simulink library "adeye_lib"  (R2019a)
settings: Solver=VariableStepAuto  StartTime=0.0  StopTime=10.0  RelTol=1e-3
undefined symbols (not defined in the file): AngularVelocity, Clock_, Data, Data_SL_Info, DiscIntNeverNeededParam, Encoding, Encoding_SL_Info, Header, Height, LinearAcceleration, Orientation, Pose, Step, Twist, Width
libraries: robotlib x47, $bdroot x46, simulink_extras x12, dspsrcs4 x6, dspindex x6, robotcorelib x2, aerolibutil x2, PreScanSimulinkLibrary x1
(part 1 of 4)
settings Model: Creator=adeye  LastModifiedBy=adeye

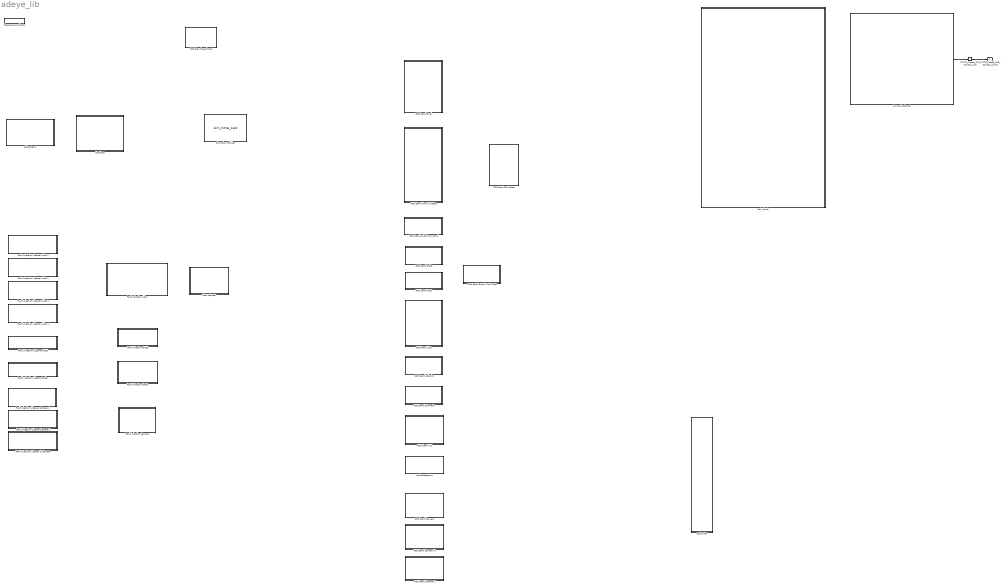
== system adeye_lib ==
  Car_Pose : Subsystem
      mask Display:
      | fprintf('Car_pose\nAdapter\n')
      | 
      | port_label('input',1,'x[m]')
      | port_label('input',2,'y[m]')
      | port_label('input',3,'z[m]')
      | port_label('input',4,'Rotx[deg]')
      | port_label('input',5,'Roty[deg]')
      | port_label('input',6,'Rotz[deg]')
      | port_label('input',7,'CoG Offset(x)')
      | port_label('input',8,'CoG Offset(y)')
      | port_label('input',9,'CoG Offset(z)')
      | 
      | port_label('output',1,'base_link_pose')
  Dynamics_Empty : Subsystem  Tag=Dynamics_Empty
  Fault Injection Camera : Subsystem  mask{idy=200, idx=100, x=100, y=150, R=0, G=0, B=0}
      mask prompts: idy "X"; idx "Y"
      mask DialogControl ParameterGroupVar Prompt: Offset
      mask DialogControl Container3 Prompt: Size
      mask DialogControl Container4 Prompt: Error
      mask Display:
      | fprintf('Fault inj\n Camera\n')
      | 
      | port_label('input',1,'R')
      | port_label('input',2,'G')
      | port_label('input',3,'B')
      | port_label('input',4,'On/Patch')
      | port_label('input',5,'patch/start_x')
      | port_label('input',6,'patch/start_y')
      | port_label('input',7,'patch/size_x')
      | port_label('input',8,'patch/size_y')
      | port_label('input',9,'patch/R')
      | port_label('input',10,'patch/G')
      | port_label('input',11,'patch/B')
      | 
      | port_label('output',1,'R')
      | port_label('output',2,'G')
      | port_label('output',3,'B')
  Fault Injection GNSS : Subsystem  mask{f=20}
      mask prompts: f "Frequency"
      mask Display:
      | fprintf('Fault inj\n GNSS\n')
      | 
      | port_label('input',1,'Pose')
      | port_label('input',2,'On/Off')
      | port_label('input',3,'noise_variance')
      | 
      | port_label('output',1,'Pose')
  Fault Injection Lidar : Subsystem  mask{f=20, p=225*16}
      mask prompts: f "Frequency"; p "Number of detection points"
      mask Display:
      | fprintf('Fault inj\n Lidar\n')
      | 
      | port_label('input',1,'Range[m]')
      | port_label('input',2,'Theta[rad]')
      | port_label('input',3,'Phi[rad]')
      | port_label('input',4,'Intensity')
      | 
      | port_label('input',5,'Off/Random/Rain')
      | 
      | port_label('input',6,'Random/range_variance')
      | port_label('input',7,'Random/theta_variance')
      | 
      | port_label('input',8,'Rain/R')
      | port_label('input',9,'Rain/a')
      | port_label('input',10,'Rain/b')
      | port_label('input',11,'Rain/p_refl_sfc')
      | port_label('input',12,'Rain/max_range')
      | 
      | port_label('output',1,'Range[m]')
      | port_label('output',2,'Theta[rad]')
      | port_label('output',3,'Phi[rad]')
      | port_label('output',4,'Intensity')
  Fault Injection Listener Camera 1 : Subsystem
      mask Display:
      | fprintf('ROS Listen Fault\n Injection Camera 1')
      | 
      | port_label('input',1,'Off/Patch')
      | port_label('input',2,'patch/start_x')
      | port_label('input',3,'patch/start_y')
      | port_label('input',4,'patch/size_x')
      | port_label('input',5,'patch/size_y')
      | port_label('input',6,'patch/R')
      | port_label('input',7,'patch/G')
      | port_label('input',8,'patch/B')
      | 
      | port_label('output',1,'Output value')
  Fault Injection Listener Camera 2 : Subsystem
      mask Display:
      | fprintf('ROS Listen Fault\n Injection Camera 2')
      | 
      | port_label('input',1,'Off/Patch')
      | port_label('input',2,'patch/start_x')
      | port_label('input',3,'patch/start_y')
      | port_label('input',4,'patch/size_x')
      | port_label('input',5,'patch/size_y')
      | port_label('input',6,'patch/R')
      | port_label('input',7,'patch/G')
      | port_label('input',8,'patch/B')
      | 
      | port_label('output',1,'Output value')
  Fault Injection Listener GNSS : Subsystem
      mask Display:
      | fprintf('ROS Listen Fault\n Injection GNSS')
      | 
      | port_label('input',1,'Off/Gaussian')
      | port_label('input',2,'noise_variance')
      | 
      | port_label('output',1,'Output value')
  Fault Injection Listener Lidar 1 : Subsystem
      mask Display:
      | fprintf('ROS Listen Fault\n Injection Lidar 1')
      | 
      | port_label('input',1,'Off/Random/Rain')
      | port_label('output',1,'Output value')
      | 
      | port_label('input',2,'Random/range_variance')
      | port_label('input',3,'Random/theta_variance')
      | 
      | port_label('input',4,'Rain/R')
      | port_label('input',5,'Rain/a')
      | port_label('input',6,'Rain/b')
      | port_label('input',7,'Rain/p_refl_sfc')
      | port_label('input',8,'Rain/max_range')
  Fault Injection Listener Lidar 2 : Subsystem
      mask Display:
      | fprintf('ROS Listen Fault\n Injection Lidar 2')
      | 
      | port_label('input',1,'Off/Random/Rain')
      | port_label('output',1,'Output value')
      | 
      | port_label('input',2,'Random/range_variance')
      | port_label('input',3,'Random/theta_variance')
      | 
      | port_label('input',4,'Rain/R')
      | port_label('input',5,'Rain/a')
      | port_label('input',6,'Rain/b')
      | port_label('input',7,'Rain/p_refl_sfc')
      | port_label('input',8,'Rain/max_range')
  Fault Injection Listener Lidar 3 : Subsystem
      mask Display:
      | fprintf('ROS Listen Fault\n Injection Lidar 3')
      | 
      | port_label('input',1,'Off/Random/Rain')
      | port_label('output',1,'Output value')
      | 
      | port_label('input',2,'Random/range_variance')
      | port_label('input',3,'Random/theta_variance')
      | 
      | port_label('input',4,'Rain/R')
      | port_label('input',5,'Rain/a')
      | port_label('input',6,'Rain/b')
      | port_label('input',7,'Rain/p_refl_sfc')
      | port_label('input',8,'Rain/max_range')
  Fault Injection Listener Lidar 4 : Subsystem
      mask Display:
      | fprintf('ROS Listen Fault\n Injection Lidar 4')
      | 
      | port_label('input',1,'Off/Random/Rain')
      | port_label('output',1,'Output value')
      | 
      | port_label('input',2,'Random/range_variance')
      | port_label('input',3,'Random/theta_variance')
      | 
      | port_label('input',4,'Rain/R')
      | port_label('input',5,'Rain/a')
      | port_label('input',6,'Rain/b')
      | port_label('input',7,'Rain/p_refl_sfc')
      | port_label('input',8,'Rain/max_range')
  Fault Injection Listener Radar : Subsystem
      mask Display:
      | fprintf('ROS Listen Fault\n Injection Radar')
      | 
      | port_label('input',1,'Off/Gaussian')
      | port_label('input',2,'range_variance')
      | port_label('input',3,'range_variance')
      | port_label('input',4,'phi_variance')
      | 
      | port_label('output',1,'Output value')
  Fault Injection Listener TL Camera : Subsystem
      mask Display:
      | fprintf('ROS Listen Fault\n Injection TL Camera')
      | 
      | port_label('input',1,'Off/Patch')
      | port_label('input',2,'patch/start_x')
      | port_label('input',3,'patch/start_y')
      | port_label('input',4,'patch/size_x')
      | port_label('input',5,'patch/size_y')
      | port_label('input',6,'patch/R')
      | port_label('input',7,'patch/G')
      | port_label('input',8,'patch/B')
      | 
      | port_label('output',1,'Output value')
  Fault Injection Radar : Subsystem  mask{n=7}
      mask prompts: n "Max number of detections of the radar"
      mask Display:
      | fprintf('Fault inj\n Radar\n')
      | 
      | port_label('input',1,'Range[m]')
      | port_label('input',2,'Theta[deg]')
      | port_label('input',3,'Phi[deg]')
      | port_label('input',4,'TargetTypeID')
      | port_label('input',5,'On/Off')
      | port_label('input',6,'range_variance')
      | port_label('input',7,'theta_variance')
      | port_label('input',8,'phi_variance')
      | 
      | port_label('output',1,'Range[m]')
      | port_label('output',2,'Theta[deg]')
      | port_label('output',3,'Phi[deg]')
      | port_label('output',4,'TargetTypeID')
  Lidar Adapter : Subsystem
      mask Display:
      | fprintf('Lidar Adapter\n')
      | 
      | port_label('input',1,'Orientation')
      | port_label('input',2,'Range[m]')
      | port_label('input',3,'Theta[rad]')
      | port_label('input',4,'Phi[rad]')
      | port_label('input',5,'Intensity')
      | 
      | port_label('output',1,'L')
  Main_block : Subsystem
  ROS Send Camera : Subsystem
      mask Display:
      | fprintf('ROS Send\n Camera 1\n')
      | 
      | port_label('input',1,'R')
      | port_label('input',2,'G')
      | port_label('input',3,'B')
  ROS Send Camera 2 : Subsystem
      mask Display:
      | fprintf('ROS Send\n Camera 2\n')
      | 
      | port_label('input',1,'R')
      | port_label('input',2,'G')
      | port_label('input',3,'B')
  ROS Send Camera TL : Subsystem
      mask Display:
      | fprintf('ROS Send\n Camera TL\n')
      | 
      | port_label('input',1,'R')
      | port_label('input',2,'G')
      | port_label('input',3,'B')
  ROS Send Clock : Subsystem  Priority=1
      mask Display:
      | fprintf('ROS Send\n Clock\n')
      | 
      | port_label('input',1,'T')
  ROS Send GNSS : Subsystem
      mask Display:
      | fprintf('ROS Send\n GNSS\n')
      | 
      | port_label('input',1,'Pose')
  ROS Send Goal : Subsystem  TreatAsAtomicUnit=on
      mask Display:
      | fprintf('ROS Send\n Goal\n')
      | 
      | port_label('input',1,'Position.x')
      | port_label('input',2,'Position.y')
      | port_label('input',3,'Position.z')
      | port_label('input',4,'Orientation.w')
      | port_label('input',5,'Orientation.x')
      | port_label('input',6,'Orientation.y')
      | port_label('input',7,'Orientation.z')
  ROS Send Groud Truth Pose : Subsystem
      mask Display:
      | fprintf('ROS Send\n Ground Truth Pose\n')
      | 
      | port_label('input',1,'Pose')
  ROS Send IMU : Subsystem
      mask Display:
      | fprintf('ROS Send\n IMU\n')
      | 
      | port_label('input',1,'Rot X [deg]')
      | port_label('input',2,'Rot Y [deg]')
      | port_label('input',3,'Rot Z [deg]')
      | port_label('input',4,'Yaw rate [m/s]')
      | port_label('input',5,'Velocity [m/s]')
  ROS Send Lidar : Subsystem
      mask Display:
      | fprintf('ROS Send\n Lidar\n')
      | 
      | port_label('input',1,'L1')
      | port_label('input',2,'L2')
      | port_label('input',3,'L3')
      | port_label('input',4,'L4')
  ROS Send Odometry : Subsystem
      mask Display:
      | fprintf('ROS Send\n Odometry\n')
      | 
      | port_label('input',1,'Pose')
      | port_label('input',2,'Velocity [m/s]')
      | port_label('input',3,'Yaw rate [m/s]')
  ROS Send Simulink State : Subsystem  TreatAsAtomicUnit=on
      mask Display:
      | fprintf('ROS Send\n Simulink State\n')
      | 
      | port_label('input',1,'Recording')
      | port_label('input',2,'Map')
      | port_label('input',3,'Sensing')
      | port_label('input',4,'Localization')
      | port_label('input',5,'Fake localization')
      | port_label('input',6,'Detection')
      | port_label('input',7,'Mission Planning')
      | port_label('input',8,'Motion Planning')
      | port_label('input',9,'Switch')
      | port_label('input',10,'Ssmp')
      | port_label('input',11,'Rviz')
  ROS Send Switch Command : Subsystem
      mask Display:
      | fprintf('ROS Send\n Switch\nCommand')
      | 
      | port_label('input',1,'S')
  ROS Send Velocity : Subsystem
      mask Display:
      | fprintf('ROS Send\n Velocity\n')
      | 
      | port_label('input',1,'V')
      | port_label('input',2,'Yaw rate')
  ROS Stop Experiment : Subsystem
      mask Display: fprintf('ROS Stop Experiment')
  ROS send RCV states : Subsystem
      mask Display:
      | fprintf('ROS send RCV states\n\n\n\n')
      | 
      | port_label('input',1,'Initial checks')
      | port_label('input',2,'Activation request')
      | port_label('input',3,'Fault')
  S-Function Builder : S-Function  InitFcn=try, set_param(gcb,'FunctionName','sim_time_calc'), end  FunctionName=sim_time_calc  SFunctionModules=sim_time_calc_wrapper  SFunctionDeploymentMode=off  EnableBusSupport=off  mask(S-Function Builder){}
      mask help: Simulink:masks:SFunctionBuilder_MD
      mask init:
      | val = [[.9  0.75 0.75 1 1 .9 .9 1]',[1 1 0.75 0.75 .9 .9 1 .9]'];try , sys = get_param(gcb,'SfunBuilderFcnName');if isempty(sys), sys = get_param(gcb,'FunctionName'); end,catch, sys = get_param(gcb,'FunctionName'); end
      settings: CopyFcn=set_param(gcbh,'LinkStatus','none')  PreSaveFcn=try, set_param(gcb,'FunctionName','sim_time_calc'), end  OpenFcn=sfunctionwizard(gcbh)
      mask Display:
      | plot(val(:,1),val(:,2))
      | disp(sys)
  STATE_Mazda_RX8_Coupe_1_rc2 : RateTransition  Tag=mux_rc/StatePort  OutPortSampleTimeOpt=Inherit
  Subsystem1 : Subsystem
      mask Display:
      | fprintf('Minimalistic Dynamics\n\n')
      | 
      | port_label('input',1,'velocity[m/s]')
      | 
      | port_label('output',1,'dx [m/s]')
      | port_label('output',2,'dy [m/s]')
      | port_label('output',3,'dz [m/s]')
      | port_label('output',4,'R [rad]')
      | port_label('output',5,'P [rad]')
      | port_label('output',6,'Y [rad]')
  frequency_evaluator : Subsystem
  pcd_writer : Subsystem
      mask Display:
      | fprintf('PCD\n Writer')
      | 
      | port_label('input',1,'X1')
      | port_label('input',2,'Y1')
      | port_label('input',3,'Z1')
      | port_label('input',4,'I1')
      | 
      | port_label('input',5,'X2')
      | port_label('input',6,'Y2')
      | port_label('input',7,'Z2')
      | port_label('input',8,'I2')
      | 
      | port_label('input',9,'X3')
      | port_label('input',10,'Y3')
      | port_label('input',11,'Z3')
      | port_label('input',12,'I3')
      | 
      | port_label('input',13,'X4')
      | port_label('input',14,'Y4')
      | port_label('input',15,'Z4')
      | port_label('input',16,'I4')
  radarDetections : Subsystem
      mask Display:
      | fprintf('ROS Send\n Radar\n')
      | 
      | port_label('input',1,'Range[m]')
      | port_label('input',2,'Theta[deg]')
      | port_label('input',3,'Phi[deg]')
      | port_label('input',4,'TargetTypeID')
  STATE_Mazda_RX8_Coupe_1_bus3 : Outport  Tag=outport/StatePort  OutDataTypeStr=Bus: PRESCAN_STATEACTUATORDATA  PortDimensions=1  SampleTime=1/20
  wires:
  Dynamics_Empty/1(State) -> STATE_Mazda_RX8_Coupe_1_rc2/1
  STATE_Mazda_RX8_Coupe_1_rc2/1 -> STATE_Mazda_RX8_Coupe_1_bus3/1

== system adeye_lib/Car_Pose ==
  note: Centering the frame in the middle of the back wheels
  x : Inport
  y : Inport  Port=2
  z : Inport  Port=3
  rot x : Inport  Port=4
  rot y : Inport  Port=5
  rot z : Inport  Port=6
  cog offset x : Inport  Port=7
  cog offset y : Inport  Port=8
  cog offset z : Inport  Port=9
  Add1 : Sum
  Add2 : Sum
  Add3 : Sum
  Coordinate Transformation Conversion : robotcorelib/Coordinate Transformation Conversion  InputRepresentation=Euler Angles  InputEulerSequence=XYZ  ShowTrVecInputPort=on  OutputRepresentation=Quaternion  OutputEulerSequence=ZYX  ShowTrVecOutputPort=on  SimulateUsing=Interpreted execution
      settings: SourceProductBaseCode=RO
  Data Type Conversion{,1..2,4} (4 alike) : DataTypeConversion
  Degrees to Radians1 : simulink_extras/Transformations/Degrees to Radians
  Degrees to Radians2 : simulink_extras/Transformations/Degrees to Radians
  Degrees to Radians5 : simulink_extras/Transformations/Degrees to Radians
  Demux : Demux  Outputs=7
  Demux1 : Demux  Outputs=3
  Mux : Mux
  Mux1 : Mux
  Mux2 : Mux
  Quaternion Conjugate1 : aerolibutil/Quaternion Conjugate
      settings: SourceProductName=Aerospace Blockset  SourceProductBaseCode=AE
  Quaternion Rotation : aerolibutil/Quaternion Rotation
  Vector Concatenate2 : Concatenate  NumInputs=3
  Vector Concatenate3 : Concatenate  NumInputs=3
  base_link_pose : Outport
  wires:
  Degrees to Radians1/1 -> Vector Concatenate2/2
  Degrees to Radians5/1 -> Vector Concatenate2/1
  Vector Concatenate2/1 -> Coordinate Transformation Conversion/1
  Degrees to Radians2/1 -> Vector Concatenate2/3
  x/1 -> Data Type Conversion/1
  y/1 -> Data Type Conversion1/1
  z/1 -> Data Type Conversion2/1
  rot x/1 -> Degrees to Radians5/1
  rot y/1 -> Degrees to Radians1/1
  rot z/1 -> Degrees to Radians2/1
  Data Type Conversion/1 -> Mux/1
  Data Type Conversion1/1 -> Mux/2
  Data Type Conversion2/1 -> Mux/3
  Coordinate Transformation Conversion/1 -> Mux/4
  Quaternion Conjugate1/1 -> Quaternion Rotation/1
  Demux/3 -> Add3/1
  Mux/1 -> Demux/1
  Quaternion Rotation/1 -> Data Type Conversion4/1
  Demux1/3 -> Add3/2
  Demux/2 -> Add2/1
  cog offset x/1 -> Vector Concatenate3/1
  Demux/7 -> Mux1/4
  Demux1/1 -> Add1/2
  Demux1/2 -> Add2/2
  Demux/4 -> Mux1/1
  Vector Concatenate3/1 -> Quaternion Rotation/2
  Add1/1 -> Mux2/1
  Mux1/1 -> Quaternion Conjugate1/1, Mux2/4
  Demux/1 -> Add1/1
  cog offset z/1 -> Vector Concatenate3/3
  cog offset y/1 -> Vector Concatenate3/2
  Demux/6 -> Mux1/3
  Mux2/1 -> base_link_pose/1
  Demux/5 -> Mux1/2
  Add3/1 -> Mux2/3
  Add2/1 -> Mux2/2
  Data Type Conversion4/1 -> Demux1/1

== system adeye_lib/Dynamics_Empty ==
  SELF_Demux_1 : Inport
  SELF_Demux_2 : Inport  Port=2
  SELF_Demux_3 : Inport  Port=3
  SELF_Demux_4 : Inport  Port=4
  SELF_Demux_5 : Inport  Port=5
  SELF_Demux_6 : Inport  Port=6
  SELF_Demux_7 : Inport  Port=7
  SELF_Demux_8 : Inport  Port=8
  SELF_Demux_9 : Inport  Port=9
  SELF_Demux_10 : Inport  Port=10
  SELF_Demux_11 : Inport  Port=11
  SELF_Demux_12 : Inport  Port=12
  MuxState : Subsystem  Tag=mux/State  mask(Empty Dynamics State Block){positioningmode=off, TimeStep=1/20}
      mask prompts: positioningmode "Positioning Mode"; TimeStep "Auto Assigned: Time Step [s]"
      mask help:
      | Build the state of an actor based on user input.
      | The user can either use positioning mode or dynamics mode.
      | - When using positioning mode the position and orientation of the actor are set directly based on the input. Expected input is relative to the initial position and orientation of the actor. It's also possible to specify the velocity of the actor, though this input isn't used, only passed on.
      | - When using dynamics mode the position input is ignored. Expected input is velocity and orientation. The velocity is relative the current orientation of the actor, while orientation is relative to its initial orientation. The position of the actor is calculated based on the velocity and orientation given.
      settings: DeleteFcn=PreScanBlockDeleteFcn;
  Subsystem1 : $bdroot/Subsystem1  SystemSampleTime=-1
  State : Outport  Tag=outport/StateOutport  SampleTime=1/20
  wires:
  SELF_Demux_10/1 -> Subsystem1/1
  Subsystem1/6 -> MuxState/9(Y [rad])
  Subsystem1/5 -> MuxState/8(P [rad])
  Subsystem1/4 -> MuxState/7(R [rad])
  Subsystem1/3 -> MuxState/6(dz [m/s])
  Subsystem1/2 -> MuxState/5(dy [m/s])
  Subsystem1/1 -> MuxState/4(dx [m/s])
  SELF_Demux_5/1 -> ?
  SELF_Demux_3/1 -> ?
  SELF_Demux_4/1 -> ?
  SELF_Demux_7/1 -> ?
  SELF_Demux_9/1 -> ?
  SELF_Demux_8/1 -> ?
  SELF_Demux_11/1 -> ?
  SELF_Demux_6/1 -> ?
  SELF_Demux_12/1 -> ?
  SELF_Demux_2/1 -> ?
  SELF_Demux_1/1 -> ?

== system adeye_lib/Fault Injection Camera ==
  In4 : Inport
  In5 : Inport  Port=2  OutDataTypeStr=uint8
  In6 : Inport  Port=3  OutDataTypeStr=uint8
  In7 : Inport  Port=4
  In1 : Inport  Port=5
  In2 : Inport  Port=6
  In3 : Inport  Port=7
  In8 : Inport  Port=8
  In9 : Inport  Port=9
  In10 : Inport  Port=10
  In11 : Inport  Port=11
  If : If
  If Action Subsystem : Subsystem  TreatAsAtomicUnit=on
  If Action Subsystem1 : Subsystem  TreatAsAtomicUnit=on
  Merge : Merge
  Merge1 : Merge
  Merge2 : Merge
  Out1 : Outport
  Out2 : Outport  Port=2
  Out3 : Outport  Port=3
  wires:
  Merge2/1 -> Out3/1
  Merge1/1 -> Out2/1
  If Action Subsystem/3(Out3) -> Merge2/1
  If Action Subsystem/2(Out2) -> Merge1/1
  If Action Subsystem/1(Out1) -> Merge/1
  Merge/1 -> Out1/1
  If Action Subsystem1/3(Output_image_B) -> Merge2/2
  If Action Subsystem1/2(Output_image_G) -> Merge1/2
  If Action Subsystem1/1(Output_image_R) -> Merge/2
  In6/1 -> If Action Subsystem1/3(image_B), If Action Subsystem/3(In3)
  In5/1 -> If Action Subsystem1/2(image_G), If Action Subsystem/2(In2)
  In4/1 -> If Action Subsystem1/1(image_R), If Action Subsystem/1(In1)
  In7/1 -> If/1
  If/2 -> If Action Subsystem/Action
  If/1 -> If Action Subsystem1/Action
  In3/1 -> If Action Subsystem1/6(size_x)
  In10/1 -> If Action Subsystem1/9(patch_G)
  In11/1 -> If Action Subsystem1/10(patch_B)
  In9/1 -> If Action Subsystem1/8(patch_R)
  In8/1 -> If Action Subsystem1/7(size_y)
  In2/1 -> If Action Subsystem1/5(start_y)
  In1/1 -> If Action Subsystem1/4(start_x)

== system adeye_lib/Fault Injection GNSS ==
  In1 : Inport
  on/off : Inport  Port=2
  noise_variance : Inport  Port=3
  If : If
  If Action Subsystem : Subsystem  TreatAsAtomicUnit=on
  If Action Subsystem1 : Subsystem  TreatAsAtomicUnit=on
  Merge : Merge
  Reshape2 : Reshape
  Out1 : Outport
  wires:
  Reshape2/1 -> If Action Subsystem/1(In1), If Action Subsystem1/1(In1)
  Merge/1 -> Out1/1
  If Action Subsystem/1(Out1) -> Merge/1
  If Action Subsystem1/1(Out1) -> Merge/2
  on/off/1 -> If/1
  In1/1 -> Reshape2/1
  If/1 -> If Action Subsystem1/Action
  If/2 -> If Action Subsystem/Action
  noise_variance/1 -> If Action Subsystem1/2(noise_variance)

== system adeye_lib/Fault Injection Lidar ==
  note: 0 for no fault injection
      | 1 for just random
      | 2 for rain model
  Range : Inport
  Theta : Inport  Port=2
  Phi : Inport  Port=3
  Intensity : Inport  Port=4
  On/Random/Rain : Inport  Port=5
  In1 : Inport  Port=6
  In2 : Inport  Port=7
  In6 : Inport  Port=8
  In7 : Inport  Port=9
  In8 : Inport  Port=10
  In9 : Inport  Port=11
  In10 : Inport  Port=12
  If : If  IfExpression=u1 > 1  ElseIfExpressions=u1 > 0
  If Action Subsystem : Subsystem  TreatAsAtomicUnit=on
  If Action Subsystem1 : Subsystem  TreatAsAtomicUnit=on
  Merge{,5..7} (4 alike) : Merge  Inputs=3
  Rain Model : Subsystem  TreatAsAtomicUnit=on
  Reshape{1..4} (4 alike) : Reshape
  Out5 : Outport
  Out6 : Outport  Port=2
  Out7 : Outport  Port=3
  Out8 : Outport  Port=4
  wires:
  In6/1 -> Rain Model/3(R)
  If/1 -> Rain Model/Action
  If Action Subsystem/3(Out3) -> Merge6/1
  Merge5/1 -> Out6/1
  Merge7/1 -> Out8/1
  If Action Subsystem1/1(Out1) -> Merge/2
  If Action Subsystem/4(Out4) -> Merge7/1
  If/3 -> If Action Subsystem/Action
  Merge6/1 -> Out7/1
  Reshape1/1 -> Rain Model/8(Theta), If Action Subsystem/2(Theta), If Action Subsystem1/2(Theta)
  If Action Subsystem/1(Out1) -> Merge/1
  Merge/1 -> Out5/1
  If Action Subsystem1/4(Out4) -> Merge7/2
  If Action Subsystem/2(Out2) -> Merge5/1
  In9/1 -> Rain Model/6(p_refl_sfc)
  Intensity/1 -> Reshape4/1
  Theta/1 -> Reshape1/1
  If/2 -> If Action Subsystem1/Action
  In10/1 -> Rain Model/7(z_max)
  In8/1 -> Rain Model/5(b)
  In7/1 -> Rain Model/4("a ")
  Range/1 -> Reshape2/1
  Reshape2/1 -> Rain Model/1(z), If Action Subsystem/1(Range), If Action Subsystem1/1(Range)
  Phi/1 -> Reshape3/1
  If Action Subsystem1/2(Out2) -> Merge5/2
  Reshape4/1 -> Rain Model/2("intensity "), If Action Subsystem/4(Intensity), If Action Subsystem1/4(Intensity)
  Rain Model/4(I) -> Merge7/3
  Rain Model/1(z_p) -> Merge/3
  Rain Model/2(T) -> Merge5/3
  Rain Model/3(P) -> Merge6/3
  Reshape3/1 -> Rain Model/9(Phi), If Action Subsystem/3(Phi), If Action Subsystem1/3(Phi)
  If Action Subsystem1/3(Out3) -> Merge6/2
  On/Random/Rain/1 -> If/1
  In1/1 -> If Action Subsystem1/5(range_variance)
  In2/1 -> If Action Subsystem1/6(theta_variance)

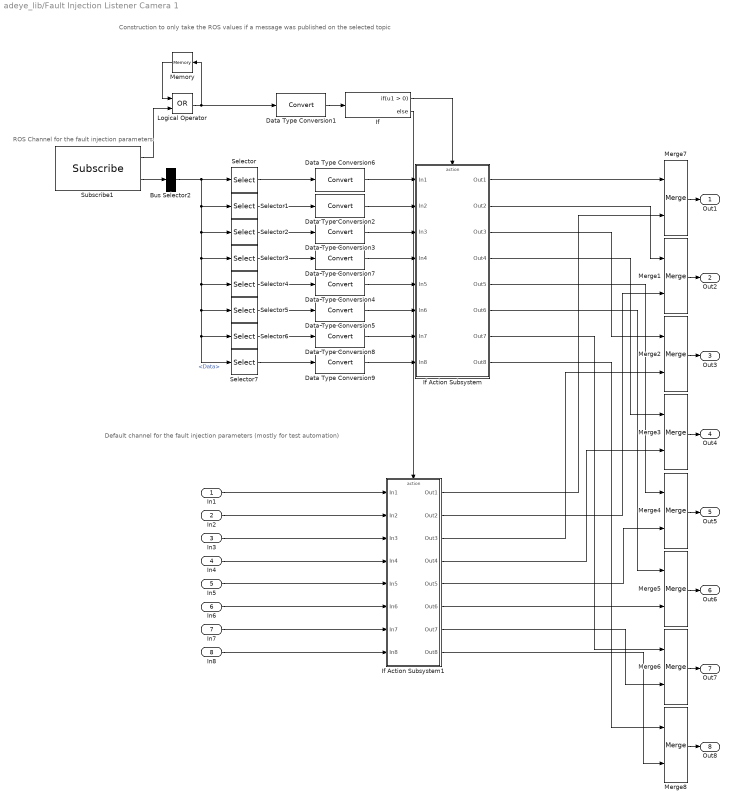
== system adeye_lib/Fault Injection Listener Camera 1 ==
  note: Default channel for the fault injection parameters (mostly for test automation)
  note: ROS Channel for the fault injection parameters
  note: Construction to only take the ROS values if a message was published on the selected topic
  In1 : Inport
  In2 : Inport  Port=2
  In3 : Inport  Port=3
  In4 : Inport  Port=4
  In5 : Inport  Port=5
  In6 : Inport  Port=6
  In7 : Inport  Port=7
  In8 : Inport  Port=8
  Bus Selector2 : BusSelector  OutputSignals=Data
  Data Type Conversion{1..9} (9 alike) : DataTypeConversion
  If : If
  If Action Subsystem : Subsystem  TreatAsAtomicUnit=on
  If Action Subsystem1 : Subsystem  TreatAsAtomicUnit=on
  Logical Operator : Logic  Operator=OR  AllPortsSameDT=off  OutDataTypeStr=boolean
  Memory : Memory  InheritSampleTime=on
  Merge{1..8} (8 alike) : Merge
  Selector : Selector  InputPortWidth=128  IndexOptions=Index vector (dialog)  Indices=[1]  OutputSizes=1
  Selector1 : Selector  InputPortWidth=128  IndexOptions=Index vector (dialog)  Indices=[2]  OutputSizes=1
  Selector2 : Selector  InputPortWidth=128  IndexOptions=Index vector (dialog)  Indices=[3]  OutputSizes=1
  Selector3 : Selector  InputPortWidth=128  IndexOptions=Index vector (dialog)  Indices=[4]  OutputSizes=1
  Selector4 : Selector  InputPortWidth=128  IndexOptions=Index vector (dialog)  Indices=[5]  OutputSizes=1
  Selector5 : Selector  InputPortWidth=128  IndexOptions=Index vector (dialog)  Indices=[6]  OutputSizes=1
  Selector6 : Selector  InputPortWidth=128  IndexOptions=Index vector (dialog)  Indices=[7]  OutputSizes=1
  Selector7 : Selector  InputPortWidth=128  IndexOptions=Index vector (dialog)  Indices=[8]  OutputSizes=1
  Subscribe1 : robotlib/Subscribe  topicSource=Specify your own  topic=/fault_injection/camera1  messageType=std_msgs/Float64MultiArray  sampleTime=-1  messageQueueLength=1
      settings: SourceProductBaseCode=RO
  Out1 : Outport
  Out2 : Outport  Port=2
  Out3 : Outport  Port=3
  Out4 : Outport  Port=4
  Out5 : Outport  Port=5
  Out6 : Outport  Port=6
  Out7 : Outport  Port=7
  Out8 : Outport  Port=8
  wires:
  If Action Subsystem/1(Out1) -> Merge7/1
  If/2 -> If Action Subsystem1/Action
  Logical Operator/1 -> Data Type Conversion1/1, Memory/1
  Subscribe1/1 -> Logical Operator/2
  Memory/1 -> Logical Operator/1
  If/1 -> If Action Subsystem/Action
  Data Type Conversion1/1 -> If/1
  If Action Subsystem1/1(Out1) -> Merge7/2
  Subscribe1/2 -> Bus Selector2/1
  In1/1 -> If Action Subsystem1/1(In1)
  Merge7/1 -> Out1/1
  Selector/1 -> Data Type Conversion6/1
  Selector7/1 -> Data Type Conversion9/1
  Selector6/1 -> Data Type Conversion8/1
  Data Type Conversion4/1 -> If Action Subsystem/5(In5)
  Selector5/1 -> Data Type Conversion5/1
  Selector3/1 -> Data Type Conversion7/1
  Data Type Conversion5/1 -> If Action Subsystem/6(In6)
  Data Type Conversion7/1 -> If Action Subsystem/4(In4)
  Data Type Conversion8/1 -> If Action Subsystem/7(In7)
  Bus Selector2/1 -> Selector7/1, Selector6/1, Selector5/1, Selector4/1, Selector3/1, Selector2/1, Selector1/1, Selector/1  "<Data>"
  Data Type Conversion9/1 -> If Action Subsystem/8(In8)
  Selector4/1 -> Data Type Conversion4/1
  Selector1/1 -> Data Type Conversion2/1
  Data Type Conversion2/1 -> If Action Subsystem/2(In2)
  Data Type Conversion6/1 -> If Action Subsystem/1(In1)
  Selector2/1 -> Data Type Conversion3/1
  Data Type Conversion3/1 -> If Action Subsystem/3(In3)
  In2/1 -> If Action Subsystem1/2(In2)
  In3/1 -> If Action Subsystem1/3(In3)
  In4/1 -> If Action Subsystem1/4(In4)
  In5/1 -> If Action Subsystem1/5(In5)
  In6/1 -> If Action Subsystem1/6(In6)
  In7/1 -> If Action Subsystem1/7(In7)
  In8/1 -> If Action Subsystem1/8(In8)
  Merge1/1 -> Out2/1
  Merge2/1 -> Out3/1
  Merge3/1 -> Out4/1
  Merge4/1 -> Out5/1
  Merge5/1 -> Out6/1
  Merge6/1 -> Out7/1
  Merge8/1 -> Out8/1
  If Action Subsystem1/8(Out8) -> Merge8/2
  If Action Subsystem1/7(Out7) -> Merge6/2
  If Action Subsystem1/6(Out6) -> Merge5/2
  If Action Subsystem1/5(Out5) -> Merge4/2
  If Action Subsystem1/4(Out4) -> Merge3/2
  If Action Subsystem1/3(Out3) -> Merge2/2
  If Action Subsystem1/2(Out2) -> Merge1/2
  If Action Subsystem/2(Out2) -> Merge1/1
  If Action Subsystem/3(Out3) -> Merge2/1
  If Action Subsystem/8(Out8) -> Merge8/1
  If Action Subsystem/4(Out4) -> Merge3/1
  If Action Subsystem/5(Out5) -> Merge4/1
  If Action Subsystem/6(Out6) -> Merge5/1
  If Action Subsystem/7(Out7) -> Merge6/1

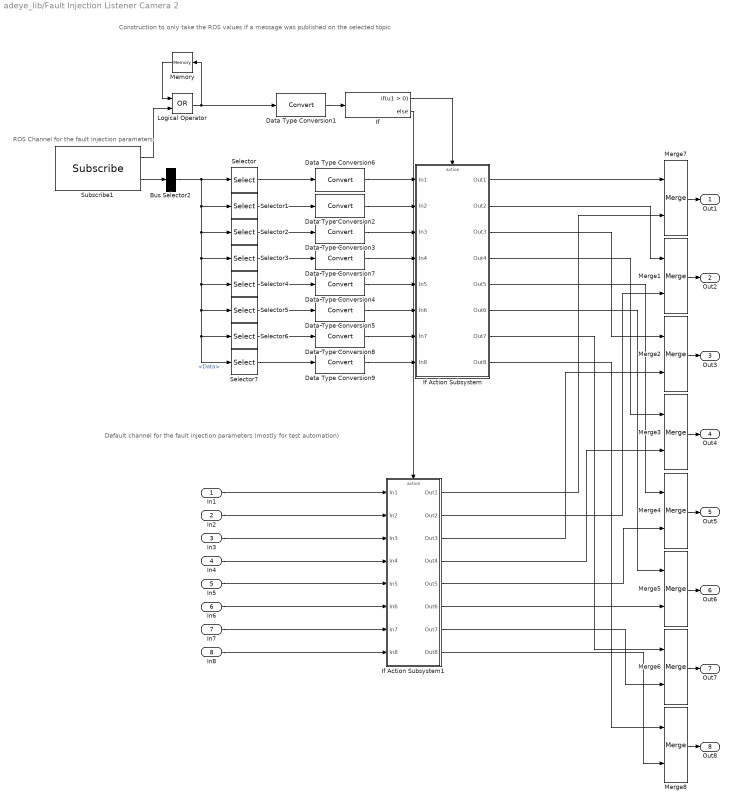
== system adeye_lib/Fault Injection Listener Camera 2 ==
  note: Default channel for the fault injection parameters (mostly for test automation)
  note: ROS Channel for the fault injection parameters
  note: Construction to only take the ROS values if a message was published on the selected topic
  In1 : Inport
  In2 : Inport  Port=2
  In3 : Inport  Port=3
  In4 : Inport  Port=4
  In5 : Inport  Port=5
  In6 : Inport  Port=6
  In7 : Inport  Port=7
  In8 : Inport  Port=8
  Bus Selector2 : BusSelector  OutputSignals=Data
  Data Type Conversion{1..9} (9 alike) : DataTypeConversion
  If : If
  If Action Subsystem : Subsystem  TreatAsAtomicUnit=on
  If Action Subsystem1 : Subsystem  TreatAsAtomicUnit=on
  Logical Operator : Logic  Operator=OR  AllPortsSameDT=off  OutDataTypeStr=boolean
  Memory : Memory  InheritSampleTime=on
  Merge{1..8} (8 alike) : Merge
  Selector : Selector  InputPortWidth=128  IndexOptions=Index vector (dialog)  Indices=[1]  OutputSizes=1
  Selector1 : Selector  InputPortWidth=128  IndexOptions=Index vector (dialog)  Indices=[2]  OutputSizes=1
  Selector2 : Selector  InputPortWidth=128  IndexOptions=Index vector (dialog)  Indices=[3]  OutputSizes=1
  Selector3 : Selector  InputPortWidth=128  IndexOptions=Index vector (dialog)  Indices=[4]  OutputSizes=1
  Selector4 : Selector  InputPortWidth=128  IndexOptions=Index vector (dialog)  Indices=[5]  OutputSizes=1
  Selector5 : Selector  InputPortWidth=128  IndexOptions=Index vector (dialog)  Indices=[6]  OutputSizes=1
  Selector6 : Selector  InputPortWidth=128  IndexOptions=Index vector (dialog)  Indices=[7]  OutputSizes=1
  Selector7 : Selector  InputPortWidth=128  IndexOptions=Index vector (dialog)  Indices=[8]  OutputSizes=1
  Subscribe1 : robotlib/Subscribe  topicSource=Specify your own  topic=/fault_injection/camera2  messageType=std_msgs/Float64MultiArray  sampleTime=-1  messageQueueLength=1
      settings: SourceProductBaseCode=RO
  Out1 : Outport
  Out2 : Outport  Port=2
  Out3 : Outport  Port=3
  Out4 : Outport  Port=4
  Out5 : Outport  Port=5
  Out6 : Outport  Port=6
  Out7 : Outport  Port=7
  Out8 : Outport  Port=8
  wires:
  If Action Subsystem/1(Out1) -> Merge7/1
  If/2 -> If Action Subsystem1/Action
  Logical Operator/1 -> Data Type Conversion1/1, Memory/1
  Subscribe1/1 -> Logical Operator/2
  Memory/1 -> Logical Operator/1
  If/1 -> If Action Subsystem/Action
  Data Type Conversion1/1 -> If/1
  If Action Subsystem1/1(Out1) -> Merge7/2
  Subscribe1/2 -> Bus Selector2/1
  In1/1 -> If Action Subsystem1/1(In1)
  Merge7/1 -> Out1/1
  Selector/1 -> Data Type Conversion6/1
  Selector7/1 -> Data Type Conversion9/1
  Selector6/1 -> Data Type Conversion8/1
  Data Type Conversion4/1 -> If Action Subsystem/5(In5)
  Selector5/1 -> Data Type Conversion5/1
  Selector3/1 -> Data Type Conversion7/1
  Data Type Conversion5/1 -> If Action Subsystem/6(In6)
  Data Type Conversion7/1 -> If Action Subsystem/4(In4)
  Data Type Conversion8/1 -> If Action Subsystem/7(In7)
  Bus Selector2/1 -> Selector7/1, Selector6/1, Selector5/1, Selector4/1, Selector3/1, Selector2/1, Selector1/1, Selector/1  "<Data>"
  Data Type Conversion9/1 -> If Action Subsystem/8(In8)
  Selector4/1 -> Data Type Conversion4/1
  Selector1/1 -> Data Type Conversion2/1
  Data Type Conversion2/1 -> If Action Subsystem/2(In2)
  Data Type Conversion6/1 -> If Action Subsystem/1(In1)
  Selector2/1 -> Data Type Conversion3/1
  Data Type Conversion3/1 -> If Action Subsystem/3(In3)
  In2/1 -> If Action Subsystem1/2(In2)
  In3/1 -> If Action Subsystem1/3(In3)
  In4/1 -> If Action Subsystem1/4(In4)
  In5/1 -> If Action Subsystem1/5(In5)
  In6/1 -> If Action Subsystem1/6(In6)
  In7/1 -> If Action Subsystem1/7(In7)
  In8/1 -> If Action Subsystem1/8(In8)
  Merge1/1 -> Out2/1
  Merge2/1 -> Out3/1
  Merge3/1 -> Out4/1
  Merge4/1 -> Out5/1
  Merge5/1 -> Out6/1
  Merge6/1 -> Out7/1
  Merge8/1 -> Out8/1
  If Action Subsystem1/8(Out8) -> Merge8/2
  If Action Subsystem1/7(Out7) -> Merge6/2
  If Action Subsystem1/6(Out6) -> Merge5/2
  If Action Subsystem1/5(Out5) -> Merge4/2
  If Action Subsystem1/4(Out4) -> Merge3/2
  If Action Subsystem1/3(Out3) -> Merge2/2
  If Action Subsystem1/2(Out2) -> Merge1/2
  If Action Subsystem/2(Out2) -> Merge1/1
  If Action Subsystem/3(Out3) -> Merge2/1
  If Action Subsystem/8(Out8) -> Merge8/1
  If Action Subsystem/4(Out4) -> Merge3/1
  If Action Subsystem/5(Out5) -> Merge4/1
  If Action Subsystem/6(Out6) -> Merge5/1
  If Action Subsystem/7(Out7) -> Merge6/1

== system adeye_lib/Fault Injection Listener GNSS ==
  note: ROS Channel for the fault injection parameters
  note: Construction to only take the ROS values if a message was published on the associated topic
  note: Default channel for the fault injection parameters (mostly for test automation)
  In1 : Inport
  In2 : Inport  Port=2
  Bus Selector2 : BusSelector  OutputSignals=Data
  Data Type Conversion1 : DataTypeConversion
  Data Type Conversion2 : DataTypeConversion
  Data Type Conversion6 : DataTypeConversion
  If : If
  If Action Subsystem : Subsystem  TreatAsAtomicUnit=on
  If Action Subsystem1 : Subsystem  TreatAsAtomicUnit=on
  Logical Operator : Logic  Operator=OR  AllPortsSameDT=off  OutDataTypeStr=boolean
  Memory : Memory  InheritSampleTime=on
  Merge1 : Merge
  Merge7 : Merge
  Selector1 : Selector  InputPortWidth=128  IndexOptions=Index vector (dialog)  Indices=[1]  OutputSizes=1
  Selector2 : Selector  InputPortWidth=128  IndexOptions=Index vector (dialog)  Indices=[2]  OutputSizes=1
  Subscribe1 : robotlib/Subscribe  topicSource=Specify your own  topic=/fault_injection/gnss  messageType=std_msgs/Float64MultiArray  sampleTime=-1  messageQueueLength=1
      settings: SourceProductBaseCode=RO
  Out1 : Outport
  Out2 : Outport  Port=2
  wires:
  Merge7/1 -> Out1/1
  In1/1 -> If Action Subsystem1/1(In1)
  Subscribe1/2 -> Bus Selector2/1
  If Action Subsystem1/1(Out1) -> Merge7/2
  Data Type Conversion1/1 -> If/1
  If/1 -> If Action Subsystem/Action
  Memory/1 -> Logical Operator/1
  Subscribe1/1 -> Logical Operator/2
  Bus Selector2/1 -> Selector2/1, Selector1/1  "<Data>"
  Logical Operator/1 -> Memory/1, Data Type Conversion1/1
  If/2 -> If Action Subsystem1/Action
  If Action Subsystem/1(Out1) -> Merge7/1
  Data Type Conversion6/1 -> If Action Subsystem/1(In1)
  Data Type Conversion2/1 -> If Action Subsystem/2(In2)
  Selector1/1 -> Data Type Conversion6/1
  Selector2/1 -> Data Type Conversion2/1
  In2/1 -> If Action Subsystem1/2(In2)
  Merge1/1 -> Out2/1
  If Action Subsystem/2(Out2) -> Merge1/1
  If Action Subsystem1/2(Out2) -> Merge1/2

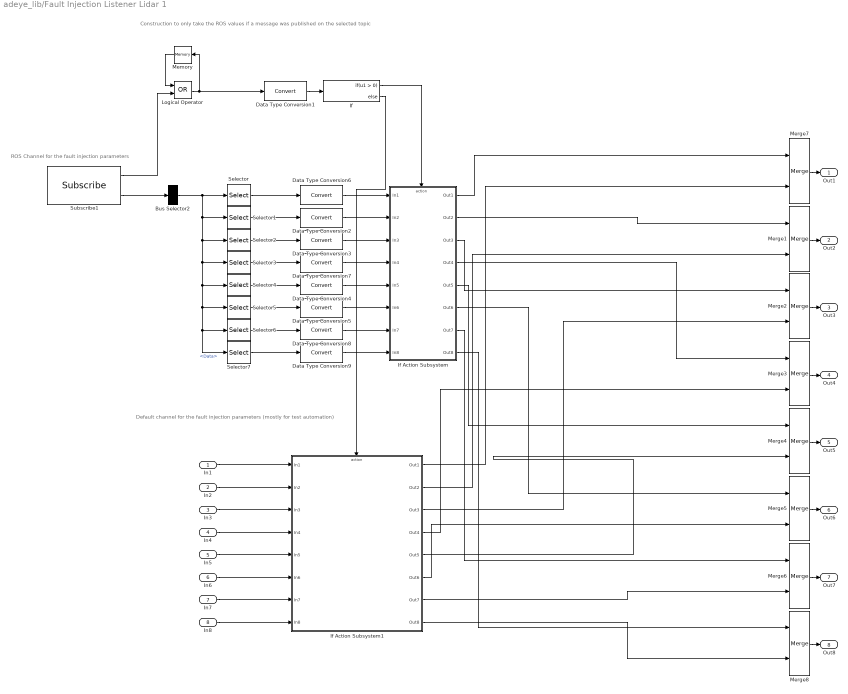
== system adeye_lib/Fault Injection Listener Lidar 1 ==
  note: Default channel for the fault injection parameters (mostly for test automation)
  note: ROS Channel for the fault injection parameters
  note: Construction to only take the ROS values if a message was published on the selected topic
  In1 : Inport
  In2 : Inport  Port=2
  In3 : Inport  Port=3
  In4 : Inport  Port=4
  In5 : Inport  Port=5
  In6 : Inport  Port=6
  In7 : Inport  Port=7
  In8 : Inport  Port=8
  Bus Selector2 : BusSelector  OutputSignals=Data
  Data Type Conversion{1..9} (9 alike) : DataTypeConversion
  If : If
  If Action Subsystem : Subsystem  TreatAsAtomicUnit=on
  If Action Subsystem1 : Subsystem  TreatAsAtomicUnit=on
  Logical Operator : Logic  Operator=OR  AllPortsSameDT=off  OutDataTypeStr=boolean
  Memory : Memory  InheritSampleTime=on
  Merge{1..8} (8 alike) : Merge
  Selector : Selector  InputPortWidth=128  IndexOptions=Index vector (dialog)  Indices=[1]  OutputSizes=1
  Selector1 : Selector  InputPortWidth=128  IndexOptions=Index vector (dialog)  Indices=[2]  OutputSizes=1
  Selector2 : Selector  InputPortWidth=128  IndexOptions=Index vector (dialog)  Indices=[3]  OutputSizes=1
  Selector3 : Selector  InputPortWidth=128  IndexOptions=Index vector (dialog)  Indices=[4]  OutputSizes=1
  Selector4 : Selector  InputPortWidth=128  IndexOptions=Index vector (dialog)  Indices=[5]  OutputSizes=1
  Selector5 : Selector  InputPortWidth=128  IndexOptions=Index vector (dialog)  Indices=[6]  OutputSizes=1
  Selector6 : Selector  InputPortWidth=128  IndexOptions=Index vector (dialog)  Indices=[7]  OutputSizes=1
  Selector7 : Selector  InputPortWidth=128  IndexOptions=Index vector (dialog)  Indices=[8]  OutputSizes=1
  Subscribe1 : robotlib/Subscribe  topicSource=Specify your own  topic=/fault_injection/lidar1  messageType=std_msgs/Float64MultiArray  sampleTime=-1  messageQueueLength=1
      settings: SourceProductBaseCode=RO
  Out1 : Outport
  Out2 : Outport  Port=2
  Out3 : Outport  Port=3
  Out4 : Outport  Port=4
  Out5 : Outport  Port=5
  Out6 : Outport  Port=6
  Out7 : Outport  Port=7
  Out8 : Outport  Port=8
  wires:
  Data Type Conversion6/1 -> If Action Subsystem/1(In1)
  If Action Subsystem/1(Out1) -> Merge7/1
  If/2 -> If Action Subsystem1/Action
  Logical Operator/1 -> Data Type Conversion1/1, Memory/1
  Subscribe1/1 -> Logical Operator/2
  Memory/1 -> Logical Operator/1
  If/1 -> If Action Subsystem/Action
  Data Type Conversion1/1 -> If/1
  If Action Subsystem1/1(Out1) -> Merge7/2
  Subscribe1/2 -> Bus Selector2/1
  In1/1 -> If Action Subsystem1/1(In1)
  Merge7/1 -> Out1/1
  Merge1/1 -> Out2/1
  Merge2/1 -> Out3/1
  Merge3/1 -> Out4/1
  Merge4/1 -> Out5/1
  Merge5/1 -> Out6/1
  Merge6/1 -> Out7/1
  Merge8/1 -> Out8/1
  If Action Subsystem/2(Out2) -> Merge1/1
  If Action Subsystem/3(Out3) -> Merge2/1
  If Action Subsystem/4(Out4) -> Merge3/1
  If Action Subsystem/5(Out5) -> Merge4/1
  If Action Subsystem/6(Out6) -> Merge5/1
  If Action Subsystem/7(Out7) -> Merge6/1
  If Action Subsystem/8(Out8) -> Merge8/1
  If Action Subsystem1/8(Out8) -> Merge8/2
  If Action Subsystem1/7(Out7) -> Merge6/2
  If Action Subsystem1/6(Out6) -> Merge5/2
  If Action Subsystem1/5(Out5) -> Merge4/2
  If Action Subsystem1/4(Out4) -> Merge3/2
  If Action Subsystem1/3(Out3) -> Merge2/2
  If Action Subsystem1/2(Out2) -> Merge1/2
  In2/1 -> If Action Subsystem1/2(In2)
  In5/1 -> If Action Subsystem1/5(In5)
  In4/1 -> If Action Subsystem1/4(In4)
  In3/1 -> If Action Subsystem1/3(In3)
  In6/1 -> If Action Subsystem1/6(In6)
  In8/1 -> If Action Subsystem1/8(In8)
  In7/1 -> If Action Subsystem1/7(In7)
  Data Type Conversion2/1 -> If Action Subsystem/2(In2)
  Selector1/1 -> Data Type Conversion2/1
  Data Type Conversion3/1 -> If Action Subsystem/3(In3)
  Selector2/1 -> Data Type Conversion3/1
  Data Type Conversion9/1 -> If Action Subsystem/8(In8)
  Data Type Conversion8/1 -> If Action Subsystem/7(In7)
  Data Type Conversion5/1 -> If Action Subsystem/6(In6)
  Data Type Conversion4/1 -> If Action Subsystem/5(In5)
  Data Type Conversion7/1 -> If Action Subsystem/4(In4)
  Selector3/1 -> Data Type Conversion7/1
  Selector4/1 -> Data Type Conversion4/1
  Selector5/1 -> Data Type Conversion5/1
  Selector6/1 -> Data Type Conversion8/1
  Selector7/1 -> Data Type Conversion9/1
  Selector/1 -> Data Type Conversion6/1
  Bus Selector2/1 -> Selector7/1, Selector6/1, Selector5/1, Selector4/1, Selector3/1, Selector2/1, Selector1/1, Selector/1  "<Data>"

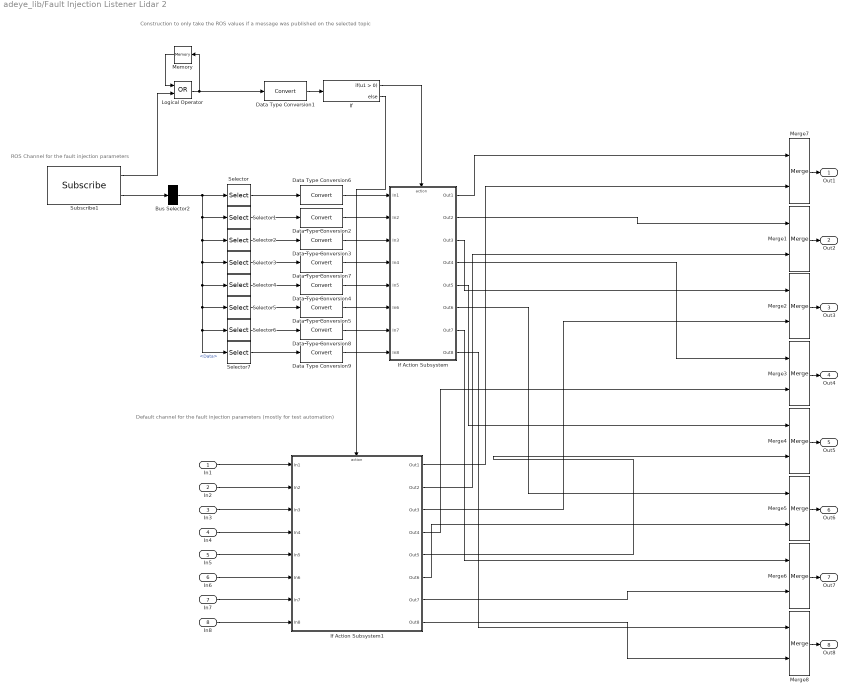
== system adeye_lib/Fault Injection Listener Lidar 2 ==
  note: Default channel for the fault injection parameters (mostly for test automation)
  note: ROS Channel for the fault injection parameters
  note: Construction to only take the ROS values if a message was published on the selected topic
  In1 : Inport
  In2 : Inport  Port=2
  In3 : Inport  Port=3
  In4 : Inport  Port=4
  In5 : Inport  Port=5
  In6 : Inport  Port=6
  In7 : Inport  Port=7
  In8 : Inport  Port=8
  Bus Selector2 : BusSelector  OutputSignals=Data
  Data Type Conversion{1..9} (9 alike) : DataTypeConversion
  If : If
  If Action Subsystem : Subsystem  TreatAsAtomicUnit=on
  If Action Subsystem1 : Subsystem  TreatAsAtomicUnit=on
  Logical Operator : Logic  Operator=OR  AllPortsSameDT=off  OutDataTypeStr=boolean
  Memory : Memory  InheritSampleTime=on
  Merge{1..8} (8 alike) : Merge
  Selector : Selector  InputPortWidth=128  IndexOptions=Index vector (dialog)  Indices=[1]  OutputSizes=1
  Selector1 : Selector  InputPortWidth=128  IndexOptions=Index vector (dialog)  Indices=[2]  OutputSizes=1
  Selector2 : Selector  InputPortWidth=128  IndexOptions=Index vector (dialog)  Indices=[3]  OutputSizes=1
  Selector3 : Selector  InputPortWidth=128  IndexOptions=Index vector (dialog)  Indices=[4]  OutputSizes=1
  Selector4 : Selector  InputPortWidth=128  IndexOptions=Index vector (dialog)  Indices=[5]  OutputSizes=1
  Selector5 : Selector  InputPortWidth=128  IndexOptions=Index vector (dialog)  Indices=[6]  OutputSizes=1
  Selector6 : Selector  InputPortWidth=128  IndexOptions=Index vector (dialog)  Indices=[7]  OutputSizes=1
  Selector7 : Selector  InputPortWidth=128  IndexOptions=Index vector (dialog)  Indices=[8]  OutputSizes=1
  Subscribe1 : robotlib/Subscribe  topicSource=Specify your own  topic=/fault_injection/lidar2  messageType=std_msgs/Float64MultiArray  sampleTime=-1  messageQueueLength=1
      settings: SourceProductBaseCode=RO
  Out1 : Outport
  Out2 : Outport  Port=2
  Out3 : Outport  Port=3
  Out4 : Outport  Port=4
  Out5 : Outport  Port=5
  Out6 : Outport  Port=6
  Out7 : Outport  Port=7
  Out8 : Outport  Port=8
  wires:
  Data Type Conversion6/1 -> If Action Subsystem/1(In1)
  If Action Subsystem/1(Out1) -> Merge7/1
  If/2 -> If Action Subsystem1/Action
  Logical Operator/1 -> Data Type Conversion1/1, Memory/1
  Subscribe1/1 -> Logical Operator/2
  Memory/1 -> Logical Operator/1
  If/1 -> If Action Subsystem/Action
  Data Type Conversion1/1 -> If/1
  If Action Subsystem1/1(Out1) -> Merge7/2
  Subscribe1/2 -> Bus Selector2/1
  In1/1 -> If Action Subsystem1/1(In1)
  Merge7/1 -> Out1/1
  Merge1/1 -> Out2/1
  Merge2/1 -> Out3/1
  Merge3/1 -> Out4/1
  Merge4/1 -> Out5/1
  Merge5/1 -> Out6/1
  Merge6/1 -> Out7/1
  Merge8/1 -> Out8/1
  If Action Subsystem/2(Out2) -> Merge1/1
  If Action Subsystem/3(Out3) -> Merge2/1
  If Action Subsystem/4(Out4) -> Merge3/1
  If Action Subsystem/5(Out5) -> Merge4/1
  If Action Subsystem/6(Out6) -> Merge5/1
  If Action Subsystem/7(Out7) -> Merge6/1
  If Action Subsystem/8(Out8) -> Merge8/1
  If Action Subsystem1/8(Out8) -> Merge8/2
  If Action Subsystem1/7(Out7) -> Merge6/2
  If Action Subsystem1/6(Out6) -> Merge5/2
  If Action Subsystem1/5(Out5) -> Merge4/2
  If Action Subsystem1/4(Out4) -> Merge3/2
  If Action Subsystem1/3(Out3) -> Merge2/2
  If Action Subsystem1/2(Out2) -> Merge1/2
  In2/1 -> If Action Subsystem1/2(In2)
  In5/1 -> If Action Subsystem1/5(In5)
  In4/1 -> If Action Subsystem1/4(In4)
  In3/1 -> If Action Subsystem1/3(In3)
  In6/1 -> If Action Subsystem1/6(In6)
  In8/1 -> If Action Subsystem1/8(In8)
  In7/1 -> If Action Subsystem1/7(In7)
  Data Type Conversion2/1 -> If Action Subsystem/2(In2)
  Selector1/1 -> Data Type Conversion2/1
  Data Type Conversion3/1 -> If Action Subsystem/3(In3)
  Selector2/1 -> Data Type Conversion3/1
  Data Type Conversion9/1 -> If Action Subsystem/8(In8)
  Data Type Conversion8/1 -> If Action Subsystem/7(In7)
  Data Type Conversion5/1 -> If Action Subsystem/6(In6)
  Data Type Conversion4/1 -> If Action Subsystem/5(In5)
  Data Type Conversion7/1 -> If Action Subsystem/4(In4)
  Selector3/1 -> Data Type Conversion7/1
  Selector4/1 -> Data Type Conversion4/1
  Selector5/1 -> Data Type Conversion5/1
  Selector6/1 -> Data Type Conversion8/1
  Selector7/1 -> Data Type Conversion9/1
  Selector/1 -> Data Type Conversion6/1
  Bus Selector2/1 -> Selector7/1, Selector6/1, Selector5/1, Selector4/1, Selector3/1, Selector2/1, Selector1/1, Selector/1  "<Data>"

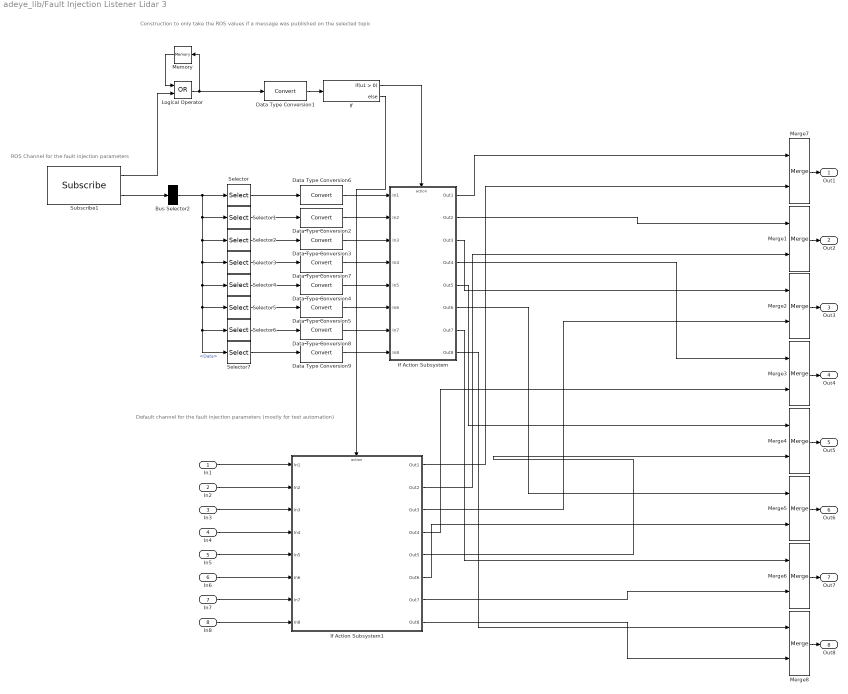
== system adeye_lib/Fault Injection Listener Lidar 3 ==
  note: Default channel for the fault injection parameters (mostly for test automation)
  note: ROS Channel for the fault injection parameters
  note: Construction to only take the ROS values if a message was published on the selected topic
  In1 : Inport
  In2 : Inport  Port=2
  In3 : Inport  Port=3
  In4 : Inport  Port=4
  In5 : Inport  Port=5
  In6 : Inport  Port=6
  In7 : Inport  Port=7
  In8 : Inport  Port=8
  Bus Selector2 : BusSelector  OutputSignals=Data
  Data Type Conversion{1..9} (9 alike) : DataTypeConversion
  If : If
  If Action Subsystem : Subsystem  TreatAsAtomicUnit=on
  If Action Subsystem1 : Subsystem  TreatAsAtomicUnit=on
  Logical Operator : Logic  Operator=OR  AllPortsSameDT=off  OutDataTypeStr=boolean
  Memory : Memory  InheritSampleTime=on
  Merge{1..8} (8 alike) : Merge
  Selector : Selector  InputPortWidth=128  IndexOptions=Index vector (dialog)  Indices=[1]  OutputSizes=1
  Selector1 : Selector  InputPortWidth=128  IndexOptions=Index vector (dialog)  Indices=[2]  OutputSizes=1
  Selector2 : Selector  InputPortWidth=128  IndexOptions=Index vector (dialog)  Indices=[3]  OutputSizes=1
  Selector3 : Selector  InputPortWidth=128  IndexOptions=Index vector (dialog)  Indices=[4]  OutputSizes=1
  Selector4 : Selector  InputPortWidth=128  IndexOptions=Index vector (dialog)  Indices=[5]  OutputSizes=1
  Selector5 : Selector  InputPortWidth=128  IndexOptions=Index vector (dialog)  Indices=[6]  OutputSizes=1
  Selector6 : Selector  InputPortWidth=128  IndexOptions=Index vector (dialog)  Indices=[7]  OutputSizes=1
  Selector7 : Selector  InputPortWidth=128  IndexOptions=Index vector (dialog)  Indices=[8]  OutputSizes=1
  Subscribe1 : robotlib/Subscribe  topicSource=Specify your own  topic=/fault_injection/lidar3  messageType=std_msgs/Float64MultiArray  sampleTime=-1  messageQueueLength=1
      settings: SourceProductBaseCode=RO
  Out1 : Outport
  Out2 : Outport  Port=2
  Out3 : Outport  Port=3
  Out4 : Outport  Port=4
  Out5 : Outport  Port=5
  Out6 : Outport  Port=6
  Out7 : Outport  Port=7
  Out8 : Outport  Port=8
  wires:
  Data Type Conversion6/1 -> If Action Subsystem/1(In1)
  If Action Subsystem/1(Out1) -> Merge7/1
  If/2 -> If Action Subsystem1/Action
  Logical Operator/1 -> Data Type Conversion1/1, Memory/1
  Subscribe1/1 -> Logical Operator/2
  Memory/1 -> Logical Operator/1
  If/1 -> If Action Subsystem/Action
  Data Type Conversion1/1 -> If/1
  If Action Subsystem1/1(Out1) -> Merge7/2
  Subscribe1/2 -> Bus Selector2/1
  In1/1 -> If Action Subsystem1/1(In1)
  Merge7/1 -> Out1/1
  Merge1/1 -> Out2/1
  Merge2/1 -> Out3/1
  Merge3/1 -> Out4/1
  Merge4/1 -> Out5/1
  Merge5/1 -> Out6/1
  Merge6/1 -> Out7/1
  Merge8/1 -> Out8/1
  If Action Subsystem/2(Out2) -> Merge1/1
  If Action Subsystem/3(Out3) -> Merge2/1
  If Action Subsystem/4(Out4) -> Merge3/1
  If Action Subsystem/5(Out5) -> Merge4/1
  If Action Subsystem/6(Out6) -> Merge5/1
  If Action Subsystem/7(Out7) -> Merge6/1
  If Action Subsystem/8(Out8) -> Merge8/1
  If Action Subsystem1/8(Out8) -> Merge8/2
  If Action Subsystem1/7(Out7) -> Merge6/2
  If Action Subsystem1/6(Out6) -> Merge5/2
  If Action Subsystem1/5(Out5) -> Merge4/2
  If Action Subsystem1/4(Out4) -> Merge3/2
  If Action Subsystem1/3(Out3) -> Merge2/2
  If Action Subsystem1/2(Out2) -> Merge1/2
  In2/1 -> If Action Subsystem1/2(In2)
  In5/1 -> If Action Subsystem1/5(In5)
  In4/1 -> If Action Subsystem1/4(In4)
  In3/1 -> If Action Subsystem1/3(In3)
  In6/1 -> If Action Subsystem1/6(In6)
  In8/1 -> If Action Subsystem1/8(In8)
  In7/1 -> If Action Subsystem1/7(In7)
  Data Type Conversion2/1 -> If Action Subsystem/2(In2)
  Selector1/1 -> Data Type Conversion2/1
  Data Type Conversion3/1 -> If Action Subsystem/3(In3)
  Selector2/1 -> Data Type Conversion3/1
  Data Type Conversion9/1 -> If Action Subsystem/8(In8)
  Data Type Conversion8/1 -> If Action Subsystem/7(In7)
  Data Type Conversion5/1 -> If Action Subsystem/6(In6)
  Data Type Conversion4/1 -> If Action Subsystem/5(In5)
  Data Type Conversion7/1 -> If Action Subsystem/4(In4)
  Selector3/1 -> Data Type Conversion7/1
  Selector4/1 -> Data Type Conversion4/1
  Selector5/1 -> Data Type Conversion5/1
  Selector6/1 -> Data Type Conversion8/1
  Selector7/1 -> Data Type Conversion9/1
  Selector/1 -> Data Type Conversion6/1
  Bus Selector2/1 -> Selector7/1, Selector6/1, Selector5/1, Selector4/1, Selector3/1, Selector2/1, Selector1/1, Selector/1  "<Data>"
